simulink model "ueb1_b"  (R2013a)
settings: Solver=ode45  StartTime=0.0  StopTime=60  RelTol=1e-3
values from neighbouring files (symbols this model uses):
  a = 0.75    [balken_parameters.m]    (also in wl_parameters_lsg.m = sqrt(2*alpha/(R*gamma)))
  A = [-alpha 1;-2*beta*x(1)*x(2)-1 beta*(1-(x(1))^2)]    [aufg32d.m]    (also in wok.m = [0,1;-om0^2,-2*dvek(i)*om0])
  ud = 0.1    [Script1_2e.m]
  y0 = [1;0]    [delta.m]
undefined symbols (not defined in the file or in its folder): B, C, D, k, y1
settings Model: Creator=isyssim2  LastModifiedBy=isyssim2

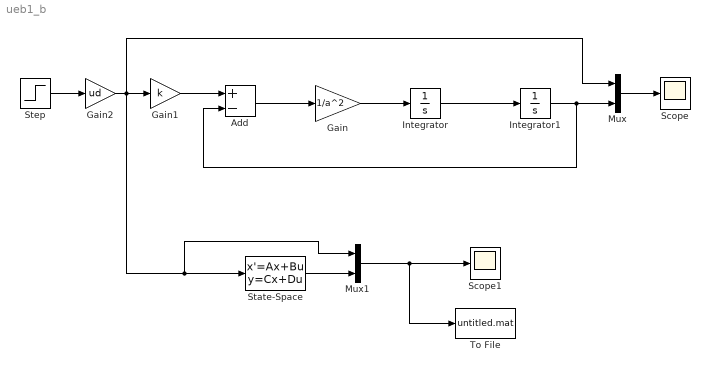
== system ueb1_b ==
  Add : Sum  Inputs=+-
  Gain : Gain  Gain=1/a^2
  Gain1 : Gain  Gain=k
  Gain2 : Gain  Gain=ud
  Integrator : Integrator  InitialCondition=y1
  Integrator1 : Integrator  InitialCondition=y0
  Mux : Mux  Inputs=2
  Mux1 : Mux  Inputs=2
  Scope : Scope
  Scope1 : Scope
  State-Space : StateSpace  A=A  B=B  C=C  D=D
  Step : Step  SampleTime=0
  To File : ToFile
  wires:
  Integrator/1 -> Integrator1/1
  Integrator1/1 -> Add/2, Mux/2
  Gain/1 -> Integrator/1
  Add/1 -> Gain/1
  Gain1/1 -> Add/1
  Step/1 -> Gain2/1
  Gain2/1 -> Mux1/1, State-Space/1, Mux/1, Gain1/1
  Mux/1 -> Scope/1
  State-Space/1 -> Mux1/2
  Mux1/1 -> To File/1, Scope1/1
